simulink model "BasicBlocksSimulink"  (R2024a)
settings: Solver=FixedStepDiscrete  StartTime=0.0  StopTime=10.0  FixedStep=0.1  RelTol=1e-3
settings Model: Creator=prabo  LastModifiedBy=prabo
settings OptimizationCC: DefaultParameterBehavior=Inlined  EnhancedBackFolding=on  PassReuseOutputArgsAs=Individual arguments  ZeroExternalMemoryAtStartup=off  ZeroInternalMemoryAtStartup=off  OptimizeBlockOrder=speed  DifferentSizesBufferReuse=on  OptimizationCustomize=off  EfficientTunableParamExpr=on
settings DebuggingCC: ParameterTunabilityLossMsg=error
settings SFSimCC: MATLABDynamicMemAlloc=off
settings RTWCC: Description=Embedded Coder  SystemTargetFile=ert.tlc  GenCodeOnly=on  TemplateMakefile=ert_default_tmf  GenerateReport=on  Toolchain=MinGW64 | gmake (64-bit Windows)  IncludeHyperlinkInReport=on  GenerateTraceInfo=on
settings CodeAppCC: ForceParamTrailComments=on  IgnoreCustomStorageClasses=off  OperatorAnnotations=on  SimulinkDataObjDesc=on  SFDataObjDesc=on  InsertBlockDesc=on
settings ERTTargetCC: TargetLangStandard=C99 (ISO)  GenerateSampleERTMain=on  CombineOutputUpdateFcns=off  InlinedParameterPlacement=NonHierarchical  ERTCustomFileTemplate=example_file_process.tlc

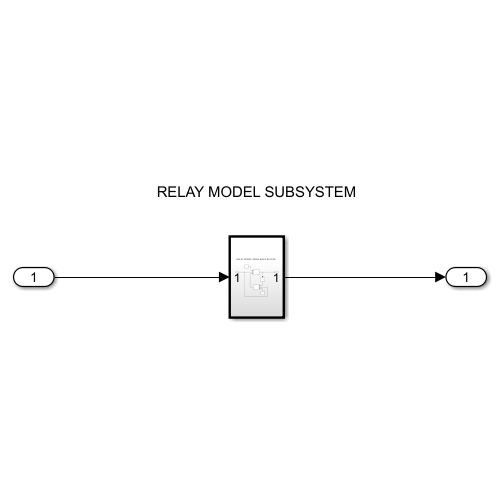
[thumbnail: Simulink's stored preview of the top-level diagram]
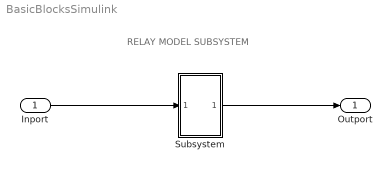
== system BasicBlocksSimulink ==
  note: RELAY MODEL SUBSYSTEM
  Inport : Inport
  Subsystem : Subsystem  TreatAsAtomicUnit=on
  Outport : Outport
  wires:
  Inport/1 -> Subsystem/1(Inport)
  Subsystem/1(Out1) -> Outport/1

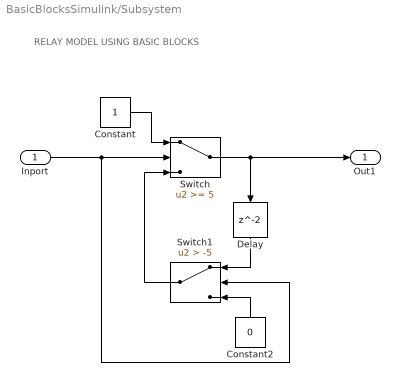
== system BasicBlocksSimulink/Subsystem ==
  note: RELAY MODEL USING BASIC BLOCKS
  Inport : Inport
  Constant : Constant
  Constant2 : Constant  Value=0
  Delay : Delay
  Switch : Switch  Threshold=5  SaturateOnIntegerOverflow=off  InputSameDT=off
  Switch1 : Switch  Criteria=u2 > Threshold  Threshold=-5  SaturateOnIntegerOverflow=off  InputSameDT=off
  Out1 : Outport
  wires:
  Switch1/1 -> Switch/3
  Switch/1 -> Delay/1, Out1/1
  Constant/1 -> Switch/1
  Constant2/1 -> Switch1/3
  Inport/1 -> Switch1/2, Switch/2
  Delay/1 -> Switch1/1
